simulink model "TestFilter"  (R2016a)
settings: Solver=FixedStepDiscrete  StartTime=0.0  StopTime=inf  FixedStep=0.02  RelTol=1e-3
settings Model: SimulationMode=external  Creator=ich  LastModifiedBy=ich
settings OptimizationCC: OptimizeModelRefInitCode=on  LifeSpan=1  MaxStackSize=64
settings HardwareCC: ProdBitPerPointer=32  ProdLargestAtomicInteger=Long  ProdLargestAtomicFloat=Double  ProdWordSize=32  ProdHWDeviceType=ARM Compatible->ARM Cortex
settings RTWCC: SystemTargetFile=ert.tlc  HardwareBoard=STM32F4-Discovery  TemplateMakefile=ert_default_tmf  GenerateReport=on  CustomInclude=MPU6050/include  Toolchain=GNU Tools for ARM Embedded Processors  IncludeHyperlinkInReport=on  LaunchReport=on  GenerateTraceInfo=on  GenerateTraceReport=on  GenerateTraceReportSl=on  GenerateTraceReportSf=on  GenerateTraceReportEml=on
settings RTWCC: CustomSource=|
  | MPU6050/source/MPU6050.c
  | MPU6050/source/stm32f4xx_i2c.c
settings CodeAppCC: ForceParamTrailComments=on  IgnoreCustomStorageClasses=off  OperatorAnnotations=on  SimulinkDataObjDesc=on  SFDataObjDesc=on  MATLABFcnDesc=on  InsertBlockDesc=on  MATLABSourceComments=on

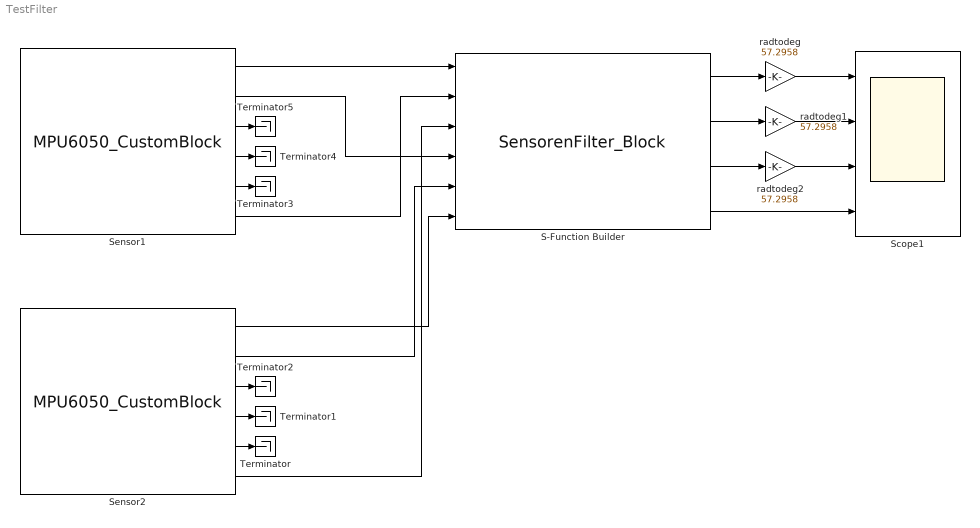
== system TestFilter ==
  S-Function Builder : S-Function  InitFcn=try, set_param(gcb,'FunctionName','SensorenFilter_Block'), end  FunctionName=SensorenFilter_Block  Parameters=single(0.02)  SFunctionModules=SensorenFilter_Block_wrapper  SFunctionDeploymentMode=off  EnableBusSupport=off  mask(S-Function Builder){}
      mask help: Simulink:masks:SFunctionBuilder_MD
      mask init:
      | val = [[.9  0.75 0.75 1 1 .9 .9 1]',[1 1 0.75 0.75 .9 .9 1 .9]'];try , sys = get_param(gcb,'SfunBuilderFcnName');if isempty(sys), sys = get_param(gcb,'FunctionName'); end,catch, sys = get_param(gcb,'FunctionName'); end
      settings: CopyFcn=set_param(gcbh,'LinkStatus','none')  PreSaveFcn=try, set_param(gcb,'FunctionName','SensorenFilter_Block'), end  OpenFcn=sfunctionwizard(gcbh)
      mask Display: plot(val(:,1),val(:,2)),disp(sys), port_label('input',1,'x1__dd'), port_label('input',2,'phi1__d'), port_label('input',3,'phi2__d'), port_label('input',4,'y1__dd'), port_label('input',5,'y2__dd'), port_label('input',6,'x2__dd'), port_label('output',1,'phi__raw'), port_label('output',2,'phi__comp'), port_label('output',3,'phi__kalman'), port_label('output',4,'phi__d')
  Scope1 : Scope  NumInputPorts=4
  Sensor1 : S-Function  InitFcn=try, set_param(gcb,'FunctionName','MPU6050_CustomBlock'), end  FunctionName=MPU6050_CustomBlock  Parameters=boolean(AD0PinLevel),uint32(LowPassBW)  SFunctionModules=MPU6050_CustomBlock_wrapper  SFunctionDeploymentMode=off  EnableBusSupport=off  mask(S-Function Builder){AD0PinLevel=0, LowPassBW=260}
      mask prompts: AD0PinLevel "Logic-Level of AD0 Pin"; LowPassBW "Low-Pass-Bandwidth [Hz]"
      mask help: Simulink:masks:SFunctionBuilder_MD
      mask init: same as TestFilter/S-Function Builder
      settings: CopyFcn=set_param(gcbh,'LinkStatus','none')  PreSaveFcn=try, set_param(gcb,'FunctionName','MPU6050_CustomBlock'), end  OpenFcn=sfunctionwizard(gcbh)
      mask TypeOptions LowPassBW: 260 | 184 | 94 | 44 | 21 | 10 | 5
      mask Display: plot(val(:,1),val(:,2)),disp(sys), port_label('output',1,'XAcceleration'), port_label('output',2,'YAcceleration'), port_label('output',3,'ZAcceleration'), port_label('output',4,'XAngularVelocity'), port_label('output',5,'YAngularVelocity'), port_label('output',6,'ZAngularVelocity')
  Sensor2 : S-Function  InitFcn=try, set_param(gcb,'FunctionName','MPU6050_CustomBlock'), end  FunctionName=MPU6050_CustomBlock  Parameters=boolean(AD0PinLevel),uint32(LowPassBW)  SFunctionModules=MPU6050_CustomBlock_wrapper  SFunctionDeploymentMode=off  EnableBusSupport=off  mask(S-Function Builder){AD0PinLevel=1, LowPassBW=260}
      mask prompts: AD0PinLevel "Logic-Level of AD0 Pin"; LowPassBW "Low-Pass-Bandwidth [Hz]"
      mask help: Simulink:masks:SFunctionBuilder_MD
      mask init: same as TestFilter/S-Function Builder
      settings: CopyFcn=set_param(gcbh,'LinkStatus','none')  PreSaveFcn=try, set_param(gcb,'FunctionName','MPU6050_CustomBlock'), end  OpenFcn=sfunctionwizard(gcbh)
      mask TypeOptions LowPassBW: 260 | 184 | 94 | 44 | 21 | 10 | 5
      mask Display: plot(val(:,1),val(:,2)),disp(sys), port_label('output',1,'XAcceleration'), port_label('output',2,'YAcceleration'), port_label('output',3,'ZAcceleration'), port_label('output',4,'XAngularVelocity'), port_label('output',5,'YAngularVelocity'), port_label('output',6,'ZAngularVelocity')
  Terminator{,1..5} (6 alike) : Terminator
  radtodeg : Gain  Gain=57.2958
  radtodeg1 : Gain  Gain=57.2958
  radtodeg2 : Gain  Gain=57.2958
  wires:
  Sensor1/3 -> Terminator5/1
  Sensor1/4 -> Terminator4/1
  Sensor1/5 -> Terminator3/1
  Sensor1/1 -> S-Function Builder/1
  Sensor1/2 -> S-Function Builder/4
  Sensor1/6 -> S-Function Builder/2
  Sensor2/1 -> S-Function Builder/6
  Sensor2/2 -> S-Function Builder/5
  Sensor2/6 -> S-Function Builder/3
  Sensor2/5 -> Terminator/1
  Sensor2/4 -> Terminator1/1
  Sensor2/3 -> Terminator2/1
  S-Function Builder/1 -> radtodeg/1
  S-Function Builder/2 -> radtodeg1/1
  S-Function Builder/3 -> radtodeg2/1
  S-Function Builder/4 -> Scope1/4
  radtodeg/1 -> Scope1/1
  radtodeg1/1 -> Scope1/2
  radtodeg2/1 -> Scope1/3
